simulink model "PLL_Sync_3_Phase"  (R2018a)
settings: Solver=ode23t  StartTime=0.0  StopTime=5  RelTol=1e-3
undefined symbols (not defined in the file): D1, Delta
libraries: powerlib x34, powerlib_meascontrol x4, simulink x3, dspswit3 x1
settings Model: Creator=samue  LastModifiedBy=samue

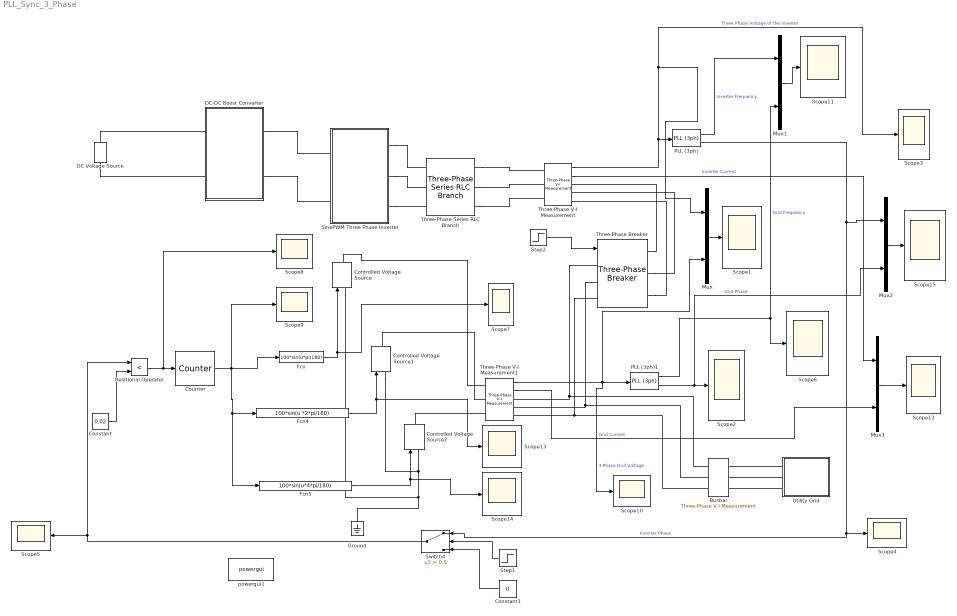
== system PLL_Sync_3_Phase ==
  Busbar : powerlib/Measurements/Three-Phase V-I Measurement  VoltageMeasurement=no  SetLabelV=off  LabelV=Vabc  Vpu=off  VpuLL=off  CurrentMeasurement=no  SetLabelI=off  LabelI=Iabc  Ipu=off  Pbase=100e6  Vbase=500e3  OutputType=Complex  PhasorSimulation=off  PSBequivalent=0
  Constant : Constant  Value=0.02
  Constant1 : Constant  Value=0
  Controlled Voltage Source : powerlib/Electrical Sources/Controlled Voltage Source  Initialize=on  Source_Type=AC  Amplitude=0  Phase=0  Frequency=60  Measurements=None
  Controlled Voltage Source1 : powerlib/Electrical Sources/Controlled Voltage Source  Initialize=on  Source_Type=AC  Amplitude=0  Phase=120  Frequency=60  Measurements=None
  Controlled Voltage Source2 : powerlib/Electrical Sources/Controlled Voltage Source  Initialize=on  Source_Type=AC  Amplitude=0  Phase=-120  Frequency=60  Measurements=None
  Counter : dspswit3/Counter  Direction=Up  CountEvent=Free running  CounterSize=User defined  MaxCount=360  InitialCount=0  Output=Count  HitValue=32  ResetInput=on  SamplesPerFrame=1  Ts=5e-5  CntDtype=double  HitDtype=Logical
  DC Voltage Source : powerlib/Electrical Sources/DC Voltage Source  Amplitude=100  Measurements=None
  DC-DC Boost Converter : Subsystem
  Fcn : Fcn  Expr=100*sin(u*pi/180)
  Fcn4 : Fcn  Expr=100*sin(u *2*pi/180)
  Fcn5 : Fcn  Expr=100*sin(u*4*pi/180)
  Ground : powerlib/Elements/Ground  LConnTagsString=a
  Mux{,1..3} (4 alike) : Mux  Inputs=2
  PLL (3ph) : powerlib_meascontrol/PLL/PLL (3ph)  Fmin=45  Par_Init=[0, 60]  ParK=[180, 3200, 1]  TcD=1e-4  MaxRateChangeFreq=12  FilterCutOffFreq=25  Ts=5e-5  AGC=on
  PLL (3ph)1 : powerlib_meascontrol/PLL/PLL (3ph)  Fmin=45  Par_Init=[0, 60]  ParK=[180, 3200, 1]  TcD=1e-4  MaxRateChangeFreq=12  FilterCutOffFreq=25  Ts=0  AGC=on
  Relational Operator : RelationalOperator  Operator=<  OutDataTypeStr=boolean  RndMeth=Simplest
  Scope{1..15} (15 alike) : Scope
  SinePWM Three Phase Inverter : Subsystem
  Step1 : Step  Time=0.06  SampleTime=0
  Step2 : Step  Time=0.1  SampleTime=0
  Switch4 : Switch  Criteria=u2 > Threshold  Threshold=0.5  RndMeth=Zero
  Three-Phase Series RLC Branch : powerlib/Elements/Three-Phase Series RLC Branch  LConnTagsString=A|B|C  RConnTagsString=A|B|C  BranchType=RLC  Resistance=1  Inductance=1e-3  Capacitance=1e-6  Measurements=None
  Three-Phase V-I Measurement : powerlib/Measurements/Three-Phase V-I Measurement  VoltageMeasurement=phase-to-ground  SetLabelV=off  LabelV=Vabc  Vpu=off  VpuLL=off  CurrentMeasurement=yes  SetLabelI=off  LabelI=Iabc  Ipu=off  Pbase=100e6  Vbase=500e3  OutputType=Complex  PhasorSimulation=off  PSBequivalent=0
  Three-Phase V-I Measurement1 : powerlib/Measurements/Three-Phase V-I Measurement  VoltageMeasurement=phase-to-ground  SetLabelV=off  LabelV=Vabc  Vpu=off  VpuLL=off  CurrentMeasurement=yes  SetLabelI=off  LabelI=Iabc  Ipu=off  Pbase=100e6  Vbase=500e3  OutputType=Complex  PhasorSimulation=off  PSBequivalent=0
  Three-Phase Breaker : powerlib/Elements/Three-Phase Breaker  InitialState=open  SwitchA=on  SwitchB=on  SwitchC=on  SwitchTimes="[1/60  5/60]"  External=on  BreakerResistance=0.01  SnubberResistance=1e6  SnubberCapacitance=inf  Measurements=None
  Utility Grid : Subsystem
  powergui1 : powerlib/powergui  Priority=1  SimulationMode=Discrete  SampleTime=5e-6  frequency=60  Iterations=50  frequencyindice=60  Pbase=100e6  ErrMax=1e-4  UnitsV=kV  UnitsW=MW  buscounter=0  FunctionMessages=off  echomessages=off  EnableUseOfTLC=off  CurrentSourceSwitches=off  DisableSnubberDevices=off  DisableRonSwitches=off  DisableVfSwitches=off  DisplayEquations=off  SolverType=Tustin/Backward Euler (TBE)  Interpol=off  ExternalGateDelay=off  methode=off  Ts=100  x0status=blocks  SPID=on  SwTol=0  HookPort=off  RestoreLinks=warning  ResistiveCurrentMeasurement=off  Frange=[0:2:500]  Ylog=off  Xlog=on  ShowGrid=off  save=off  variable=ZData  structure=0  ZoomFFT=off  StartTime=0.0  cycles=1  DisplayStyle=1  fundamental=60  FreqAxis=off  MaxFrequency=1000  frequencyindicesteady=1  RmsSteady=1  display=off
  wires:
  PLL (3ph)/2 -> Mux2/1, Switch4/1, Scope4/1  "Inverter Phase"
  Three-Phase V-I Measurement1/1 -> PLL (3ph)1/1, Mux/2, Scope10/1  "3 Phase Grid Voltage"
  Step1/1 -> Switch4/2
  Constant1/1 -> Switch4/3
  Step2/1 -> Three-Phase Breaker/1
  Three-Phase V-I Measurement/1 -> Scope3/1, Mux/1, PLL (3ph)/1  "Three Phase Voltage of the Inverter"
  Mux/1 -> Scope1/1
  PLL (3ph)1/2 -> Scope2/1, Mux2/2  "Grid Phase"
  PLL (3ph)1/1 -> Scope6/1, Mux1/2  "Grid Frequency"
  Counter/1 -> Scope9/1, Fcn/1, Fcn5/1, Fcn4/1
  Fcn/1 -> Scope7/1, Controlled Voltage Source/1
  Fcn5/1 -> Scope14/1, Controlled Voltage Source2/1
  Relational Operator/1 -> Scope8/1, Counter/1
  Constant/1 -> Relational Operator/2
  Switch4/1 -> Scope5/1, Relational Operator/1
  Fcn4/1 -> Scope13/1, Controlled Voltage Source1/1
  Mux1/1 -> Scope11/1
  PLL (3ph)/1 -> Mux1/1  "Inverter Frequency"
  Mux2/1 -> Scope15/1
  Three-Phase V-I Measurement/2 -> Mux3/1  "Inverter Current"
  Three-Phase V-I Measurement1/2 -> Mux3/2  "Grid Current"
  Mux3/1 -> Scope12/1
  connections:
  Three-Phase Breaker/RConn3 -- Three-Phase V-I Measurement/RConn3
  Three-Phase Breaker/RConn2 -- Three-Phase V-I Measurement/RConn2
  Three-Phase Breaker/RConn1 -- Three-Phase V-I Measurement/RConn1
  Three-Phase Breaker/LConn3 -- Busbar/LConn3 -- Three-Phase V-I Measurement1/RConn3
  Three-Phase Breaker/LConn2 -- Busbar/LConn2 -- Three-Phase V-I Measurement1/RConn2
  Three-Phase Breaker/LConn1 -- Busbar/LConn1 -- Three-Phase V-I Measurement1/RConn1
  Ground/LConn1 -- Controlled Voltage Source/LConn1 -- Controlled Voltage Source1/LConn1 -- Controlled Voltage Source2/LConn1
  Controlled Voltage Source/RConn1 -- Three-Phase V-I Measurement1/LConn1
  Controlled Voltage Source1/RConn1 -- Three-Phase V-I Measurement1/LConn2
  Controlled Voltage Source2/RConn1 -- Three-Phase V-I Measurement1/LConn3
  Three-Phase Series RLC Branch/RConn1 -- Three-Phase V-I Measurement/LConn1
  Three-Phase Series RLC Branch/RConn2 -- Three-Phase V-I Measurement/LConn2
  Three-Phase Series RLC Branch/RConn3 -- Three-Phase V-I Measurement/LConn3
  SinePWM Three Phase Inverter/RConn1 -- Three-Phase Series RLC Branch/LConn1
  SinePWM Three Phase Inverter/RConn2 -- Three-Phase Series RLC Branch/LConn2
  SinePWM Three Phase Inverter/RConn3 -- Three-Phase Series RLC Branch/LConn3
  Utility Grid/LConn1 -- Busbar/RConn1
  Utility Grid/LConn2 -- Busbar/RConn2
  Utility Grid/LConn3 -- Busbar/RConn3
  DC Voltage Source/LConn1 -- DC-DC Boost Converter/LConn2
  DC Voltage Source/RConn1 -- DC-DC Boost Converter/LConn1
  DC-DC Boost Converter/RConn1 -- SinePWM Three Phase Inverter/LConn1
  DC-DC Boost Converter/RConn2 -- SinePWM Three Phase Inverter/LConn2

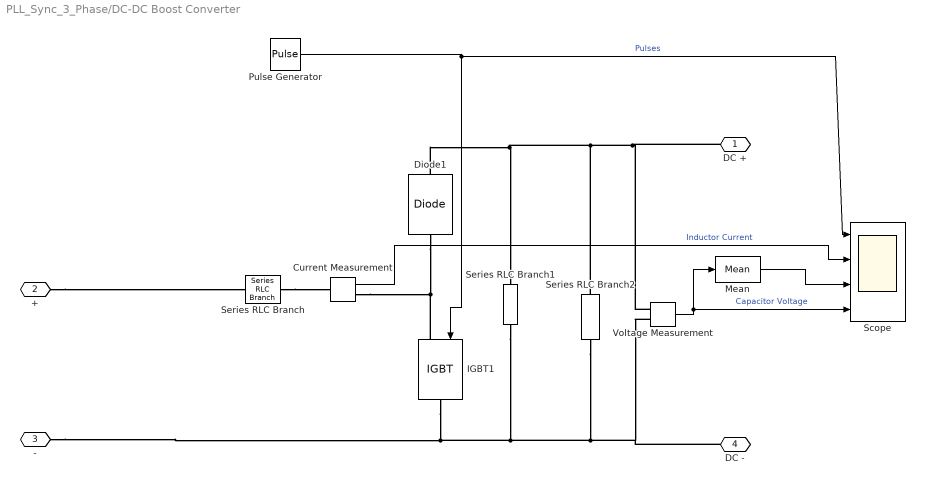
== system PLL_Sync_3_Phase/DC-DC Boost Converter ==
  Current Measurement : powerlib/Measurements/Current Measurement  PhasorSimulation=off  OutputType=Complex  PSBequivalent=0
  Diode1 : powerlib/Power Electronics/Diode  Ron=0.001  Lon=0  Vf=0.00001  IC=0  UseSnubber=0  Rs=5000000  Cs=250e-9  Measurements=off
  IGBT1 : powerlib/Power Electronics/IGBT  Ron=0.001  Lon=0  Vf=0.0001  Tf=1e-6  Tt=2e-6  IC=0  Rs=1e5  Cs=inf  Measurements=off
  Mean : powerlib_meascontrol/Measurements/Mean  Freq=60  Vinit=0  Ts=0
  Pulse Generator : DiscretePulseGenerator  PulseType=Time based  Period=1e-5  PulseWidth=50
  Scope : Scope  NumInputPorts=4
  Series RLC Branch : powerlib/Elements/Series RLC Branch  LConnTagsString=__new0  RConnTagsString=__new0  BranchType=L  Resistance=1  Inductance=200e-6  SetiL0=off  InitialCurrent=0  Capacitance=1e-6  Setx0=off  InitialVoltage=0  Measurements=None
  Series RLC Branch1 : powerlib/Elements/Series RLC Branch  LConnTagsString=__new0  RConnTagsString=__new0  BranchType=C  Resistance=1  Inductance=1e-3  SetiL0=off  InitialCurrent=0  Capacitance=100e-6  Setx0=off  InitialVoltage=0  Measurements=None
  Series RLC Branch2 : powerlib/Elements/Series RLC Branch  LConnTagsString=__new0  RConnTagsString=__new0  BranchType=R  Resistance=12  Inductance=1e-3  SetiL0=off  InitialCurrent=0  Capacitance=1e-6  Setx0=off  InitialVoltage=0  Measurements=None
  Voltage Measurement : powerlib/Measurements/Voltage Measurement  PhasorSimulation=off  OutputType=Complex  PSBequivalent=0
  DC + : PMIOPort  Side=Right
  + : PMIOPort  Port=2  Side=Left
  - : PMIOPort  Port=3  Side=Left
  DC - : PMIOPort  Port=4  Side=Right
  wires:
  Current Measurement/1 -> Scope/2  "Inductor Current"
  Voltage Measurement/1 -> Scope/4, Mean/1  "Capacitor Voltage"
  Pulse Generator/1 -> Scope/1, IGBT1/1  "Pulses"
  Mean/1 -> Scope/3
  connections:
  IGBT1/RConn1 -- Series RLC Branch1/RConn1 -- Voltage Measurement/LConn2 -- DC -/RConn1 -- Series RLC Branch2/RConn1 -- -/RConn1
  Voltage Measurement/LConn1 -- DC +/RConn1 -- Series RLC Branch2/LConn1 -- Diode1/RConn1 -- Series RLC Branch1/LConn1
  Diode1/LConn1 -- IGBT1/LConn1 -- Current Measurement/RConn1
  Series RLC Branch/RConn1 -- Current Measurement/LConn1
  +/RConn1 -- Series RLC Branch/LConn1

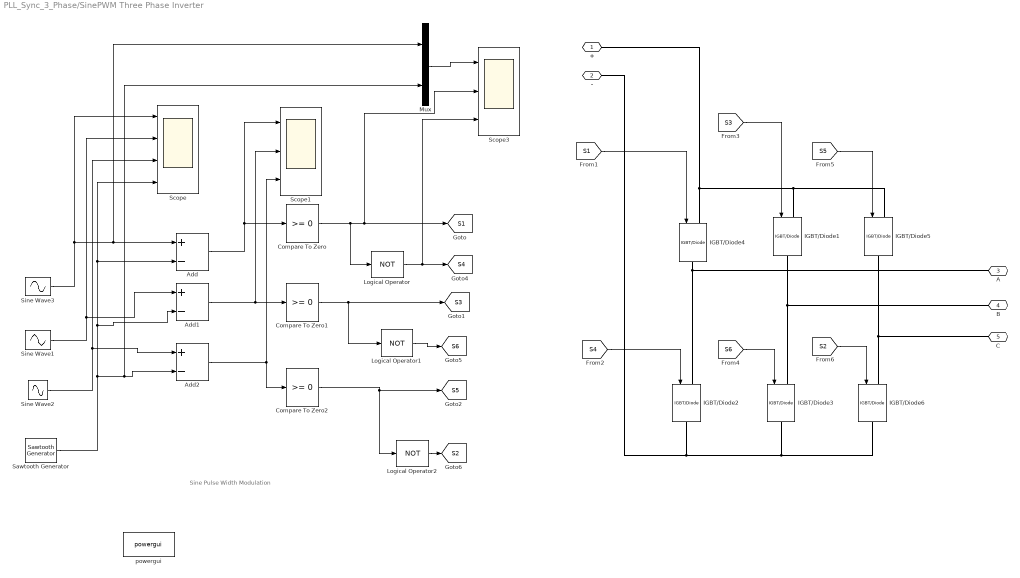
== system PLL_Sync_3_Phase/SinePWM Three Phase Inverter ==
  note: Sine Pulse Width Modulation
  Add : Sum  Inputs=+-
  Add1 : Sum  Inputs=+-
  Add2 : Sum  Inputs=+-
  Compare To Zero : simulink/Logic and Bit Operations/Compare To Zero  relop=>=  OutDataTypeStr=boolean
  Compare To Zero1 : simulink/Logic and Bit Operations/Compare To Zero  relop=>=  OutDataTypeStr=boolean
  Compare To Zero2 : simulink/Logic and Bit Operations/Compare To Zero  relop=>=  OutDataTypeStr=boolean
  IGBT/Diode{1..6} (6 alike) : powerlib/Power Electronics/IGBT//Diode  Ron=1e-3  Rs=1e5  Cs=inf  Measurements=off
  Logical Operator : Logic  Operator=NOT  AllPortsSameDT=off  OutDataTypeStr=boolean
  Logical Operator1 : Logic  Operator=NOT  AllPortsSameDT=off  OutDataTypeStr=boolean
  Logical Operator2 : Logic  Operator=NOT  AllPortsSameDT=off  OutDataTypeStr=boolean
  Mux : Mux  Inputs=2
  Sawtooth Generator : powerlib_meascontrol/Pulse & Signal Generators/Sawtooth Generator  Freq=1e3  Phase=180  Ts=0
      settings: SourceProductName=Simscape Power Systems
  Scope : Scope  NumInputPorts=4
  Scope1 : Scope  NumInputPorts=3
  Scope3 : Scope  NumInputPorts=3
  Sine Wave1 : Sin  Frequency=2*pi*60  Phase=(2*pi)/3  SampleTime=0
  Sine Wave2 : Sin  Frequency=2*pi*60  Phase=(-2*pi)/3  SampleTime=0
  Sine Wave3 : Sin  Frequency=2*pi*60  SampleTime=0
  powergui : powerlib/powergui  Priority=1  SimulationMode=Continuous  SampleTime=50e-6  frequency=60  Iterations=50  frequencyindice=0  Pbase=100e6  ErrMax=1e-4  UnitsV=kV  UnitsW=MW  buscounter=0  FunctionMessages=off  echomessages=off  EnableUseOfTLC=off  CurrentSourceSwitches=off  DisableSnubberDevices=off  DisableRonSwitches=off  DisableVfSwitches=off  DisplayEquations=off  SolverType=Tustin/Backward Euler (TBE)  Interpol=off  ExternalGateDelay=off  methode=off  Ts=100  x0status=blocks  SPID=on  SwTol=0  HookPort=off  RestoreLinks=warning  ResistiveCurrentMeasurement=off  Frange=[0:2:500]  Ylog=off  Xlog=on  ShowGrid=off  save=off  variable=ZData  structure=0  ZoomFFT=off  StartTime=0.0  cycles=1  DisplayStyle=1  fundamental=60  FreqAxis=off  MaxFrequency=1000  frequencyindicesteady=1  RmsSteady=1  display=off
  + : PMIOPort  Side=Left
  - : PMIOPort  Port=2  Side=Left
  A : PMIOPort  Port=3  Side=Right
  B : PMIOPort  Port=4  Side=Right
  C : PMIOPort  Port=5  Side=Right
  tag scope: S1=global, S2=global, S3=global, S4=global, S5=global, S6=global
  wires:
  Sawtooth Generator/1 -> Mux/2, Add2/2, Add1/2, Add/2, Scope/4
  Add/1 -> Scope1/1, Compare To Zero/1
  Add1/1 -> Compare To Zero1/1, Scope1/2
  Compare To Zero/1 -> [S1], Scope3/2, Logical Operator/1
  [S6] -> IGBT/Diode3/1
  Compare To Zero1/1 -> Logical Operator1/1, [S3]
  Sine Wave3/1 -> Mux/1, Add/1, Scope/1
  Sine Wave2/1 -> Add2/1, Scope/3
  Mux/1 -> Scope3/1
  Compare To Zero2/1 -> Logical Operator2/1, [S5]
  [S2] -> IGBT/Diode6/1
  [S1] -> IGBT/Diode4/1
  [S3] -> IGBT/Diode1/1
  [S4] -> IGBT/Diode2/1
  [S5] -> IGBT/Diode5/1
  Add2/1 -> Compare To Zero2/1, Scope1/3
  Sine Wave1/1 -> Add1/1, Scope/2
  Logical Operator2/1 -> [S2]
  Logical Operator1/1 -> [S6]
  Logical Operator/1 -> Scope3/3, [S4]
  connections:
  IGBT/Diode6/LConn1 -- C/RConn1 -- IGBT/Diode5/RConn1
  IGBT/Diode4/RConn1 -- IGBT/Diode2/LConn1 -- A/RConn1
  IGBT/Diode4/LConn1 -- +/RConn1 -- IGBT/Diode5/LConn1 -- IGBT/Diode1/LConn1
  IGBT/Diode6/RConn1 -- -/RConn1 -- IGBT/Diode2/RConn1 -- IGBT/Diode3/RConn1
  IGBT/Diode3/LConn1 -- B/RConn1 -- IGBT/Diode1/RConn1

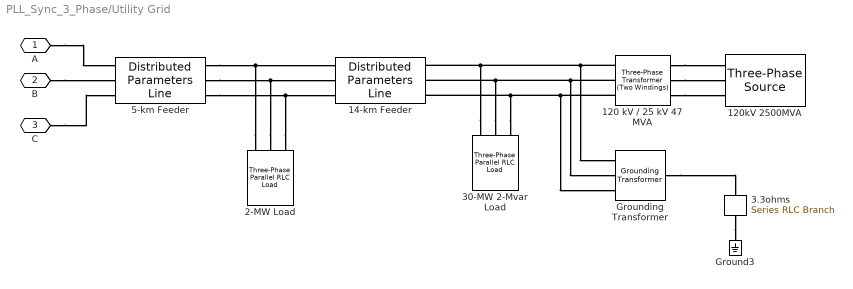
== system PLL_Sync_3_Phase/Utility Grid ==
  120 kV / 25 kV 47 MVA : powerlib/Elements/Three-Phase Transformer (Two Windings)  Winding1Connection=Yg  Winding2Connection=Delta (D1)  CoreType=Three single-phase transformers  SetSaturation=off  Hysteresis=off  DataFile='basic_model'  SetInitialFlux=off  Measurements=None  UNITS=pu  NominalPower=[47e6 60 ]  Winding1="[ 120e3  0.08/30   0.08 ]"  Winding2="[ 25e3  0.08/30  0.08]"  Rm=500  Lm=500  L0=0.5  Saturation="[ 0,0  ;  0.005,1.2  ;  1.0,1.4 ]"  InitialFluxes=[ 0.8 , -0.8 , 0.7 ]  MoreParameters=off  BreakLoop=off  DataType=off  TransfoNumber=0
  120kV 2500MVA : powerlib/Electrical Sources/Three-Phase Source  InternalConnection=Yg  VoltagePhases=off  Voltage=120e3  PhaseAngle=0  Voltage_phases=[25e3 25e3 25e3]/sqrt(3)  PhaseAngles_phases=[0 -120 +120]  Frequency=60  NonIdealSource=on  SpecifyImpedance=on  Resistance=0.8929  Inductance=16.58e-3  ShortCircuitLevel=2500e6  BaseVoltage=120e3  XRratio=7  BusType=swing  Pref=0  Qref=0  Prefabc=[10e3, 10e3, 10e3]  Qrefabc=[0, 0, 0]  Qmin=-inf  Qmax=inf
  14-km Feeder : powerlib/Elements/Distributed Parameters Line  Phases=3  Frequency=60  Resistance=[0.1153 0.413]  Inductance=[1.05e-3 3.32e-3]  Capacitance=[11.33e-009 5.01e-009]  Length=14  x1=[-6e-05 1.37030160408931e-09 -837.178421983371 -4898.29413559374;-5.5e-05 1.36683884590095e-09 -827.943873256933 -4899.86347684942;-5e-05 1.36337123125689e-09 -818.706382799107 -4901.41540861316;-4.5e-05 1.35989877247778e-09 -809.46598343122 -4902.94992537087;-4e-05 1.35642148190145e-09 -800.222707984933 -4904.46702167032;-3.5e-05 1.35293937188291e-09 -790.976589302125 -4905.96669212118;-3e-05 1.3494524547943e-09 -781.727660234781 -4907.44893139504;-2.5e-05 1.34596074302483e-09 -772.475953644866 -4908.91373422541;-2e-05 1.34246424898074e-09 -763.221502404218 -4910.36109540777;-1.5e-05 1.33896298508529e-09 -753.964339394426 -4911.79100979957;-1e-05 1.33545696377866e-09 -744.704497506712 -4913.20347232023;-5e-06 1.33194619751794e-09 -735.442009641819 -4914.59847795121]  x2=[-6e-05 5.08712230264926e-09 -3097.87964222434 -18651.9887557223;-5.5e-05 5.07453697378858e-09 -3062.7159890635 -18657.7949820346;-5e-05 5.06193361481116e-09 -3027.54145389961 -18663.5349161465;-4.5e-05 5.04931227049744e-09 -2992.35616170978 -18669.2085376637;-4e-05 5.03667298569178e-09 -2957.16023750934 -18674.8158264276;-3.5e-05 5.02401580530226e-09 -2921.95380635141 -18680.3567625152;-3e-05 5.01134077430056e-09 -2886.73699332641 -18685.8313262391;-2.5e-05 4.99864793772179e-09 -2851.50992356168 -18691.239498148;-2e-05 4.98593734066431e-09 -2816.27272222099 -18696.5812590262;-1.5e-05 4.9732090282896e-09 -2781.02551450411 -18701.8565898943;-1e-05 4.96046304582206e-09 -2745.76842564636 -18707.0654720087;-5e-06 4.94769943854889e-09 -2710.50158091816 -18712.2078868619]  x3=[-6e-05 3.12910261542347e-10 -2393.9333377164 -305.532683111771;-5.5e-05 3.1311058091873e-10 -2393.35316962759 -310.044595684322;-5e-05 3.13309787795519e-10 -2392.76449781966 -314.555406650896;-4.5e-05 3.13507881464919e-10 -2392.1673243842 -319.065099984328;-4e-05 3.13704861223094e-10 -2391.561651443 -323.573659661422;-3.5e-05 3.13900726370161e-10 -2390.94748114805 -328.081069663011;-3e-05 3.14095476210203e-10 -2390.32481568154 -332.587313974013;-2.5e-05 3.14289110051261e-10 -2389.69365725583 -337.092376583486;-2e-05 3.14481627205343e-10 -2389.05400811345 -341.596241484688;-1.5e-05 3.14673026988426e-10 -2388.40587052713 -346.098892675133;-1e-05 3.14863308720454e-10 -2387.74924679973 -350.600314156646;-5e-06 3.15052471725347e-10 -2387.08413926427 -355.100489935423]  x4=[-6e-05 -3.04931956519203e-10 2380.3561252703 228.597013568549;-5.5e-05 -3.05150318536322e-10 2379.92100153645 233.08347039212;-5e-05 -3.05367596337108e-10 2379.47742180874 237.569099056944;-4.5e-05 -3.05583789149561e-10 2379.02538766323 242.053883625328;-4e-05 -3.05798896205536e-10 2378.56490070603 246.537808162581;-3.5e-05 -3.06012916740745e-10 2378.09596257327 251.020856737063;-3e-05 -3.06225849994761e-10 2377.61857493111 255.503013420251;-2.5e-05 -3.06437695211021e-10 2377.13273947575 259.984262286788;-2e-05 -3.06648451636826e-10 2376.63845793338 264.464587414544;-1.5e-05 -3.06858118523346e-10 2376.1357320602 268.943972884669;-1e-05 -3.07066695125624e-10 2375.62456364245 273.422402781655;-5e-06 -3.07274180702576e-10 2375.10495449632 277.899861193387]  x5=5.70973484498186e-05  V1=ones(3,3)  V2=ones(3,3)  I1=ones(3,3)  I2=ones(3,3)  nHarmo=1  Measurements=None
      settings: SourceProductName=Simscape Power Systems
  2-MW Load : powerlib/Elements/Three-Phase Parallel RLC Load  LConnTagsString=A|B|C  Configuration=Y (grounded)  NominalVoltage=25e3  Vabc=[1e3 1e3 1e3]  Vabcp=[1e3 1e3 1e3]  NominalFrequency=60  UnbalancedPower=off  ActivePower=2e6  InductivePower=0  CapacitivePower=0  Pabc=[10e3 9e3 11e3]  QLabc=[100 90 110]  QCabc=[100 90 110]  Pabcp=[10e3 9e3 11e3]  QLabcp=[100 90 110]  QCabcp=[100 90 110]  Measurements=None  LoadType=constant Z
  "3.3ohms " : powerlib/Elements/Series RLC Branch  LConnTagsString=__new0  RConnTagsString=__new0  BranchType=R  Resistance=3.3  Inductance=[]  SetiL0=off  InitialCurrent=0  Capacitance=[]  Setx0=off  InitialVoltage=0  Measurements=None
  30-MW 2-Mvar Load : powerlib/Elements/Three-Phase Parallel RLC Load  LConnTagsString=A|B|C  Configuration=Y (grounded)  NominalVoltage=25e3  Vabc=[1e3 1e3 1e3]  Vabcp=[1e3 1e3 1e3]  NominalFrequency=60  UnbalancedPower=off  ActivePower=30e6  InductivePower=2e6  CapacitivePower=0  Pabc=[10e3 9e3 11e3]  QLabc=[100 90 110]  QCabc=[100 90 110]  Pabcp=[10e3 9e3 11e3]  QLabcp=[100 90 110]  QCabcp=[100 90 110]  Measurements=None  LoadType=constant Z
  5-km Feeder : powerlib/Elements/Distributed Parameters Line  Phases=3  Frequency=60  Resistance=[0.1153 0.413]  Inductance=[1.05e-3 3.32e-3]  Capacitance=[11.33e-009 5.01e-009]  Length=5  x1=[-2.5e-05 0 0 0;-2e-05 0 0 0;-1.5e-05 0 0 0;-1e-05 0 0 0;-5e-06 0 0 0]  x2=[-2.5e-05 1.34584545405026e-09 0 0;-2e-05 1.34234927961883e-09 -763.221502404218 -4910.36109540777;-1.5e-05 1.33884833574454e-09 -753.964339394426 -4911.79100979957;-1e-05 1.33534263486641e-09 -744.704497506712 -4913.20347232023;-5e-06 1.33183218944042e-09 -735.442009641819 -4914.59847795121]  x3=[-2.5e-05 3.30735135908525e-10 0 0;-2e-05 3.30933481340074e-10 -2388.24027947955 -310.379138748703;-1.5e-05 3.31130650946255e-10 -2387.65098615636 -314.880311555783;-1e-05 3.31326644026514e-10 -2387.05320937425 -319.380365575314;-5e-06 3.31521459884476e-10 -2386.44695125713 -323.879284818352]  x4=[-2.5e-05 -3.29438575094476e-10 0 0;-2e-05 -3.29640752377991e-10 2385.68435713408 294.280195880359;-1.5e-05 -3.29841758429277e-10 2385.12541412599 298.776579490401;-1e-05 -3.30041592534149e-10 2384.55799663246 303.271901530365;-5e-06 -3.30240253982584e-10 2383.98210666956 307.766146028118]  x5=2.03919101606495e-05  V1=ones(3,3)  V2=ones(3,3)  I1=ones(3,3)  I2=ones(3,3)  nHarmo=1  Measurements=None
      settings: SourceProductName=Simscape Power Systems
  Ground3 : powerlib/Elements/Ground  LConnTagsString=a
  "Grounding Transformer " : powerlib/Elements/Grounding Transformer   UNITS=pu  NominalPower="[100e6   60]"  NominalVoltage=25e3  ZeroSequenceImpedance_pu=[0.025 0.75]  MagnetizationBranch_pu=[500 500]  ZeroSequenceImpedance_SI=[0.052083 589.05]  MagnetizationBranch_SI=[1041.7 3.927e+005]  Measurements=None
      settings: SourceProductName=Simscape Power Systems  SourceProductBaseCode=PS
  A : PMIOPort  Side=Left
  B : PMIOPort  Port=2  Side=Left
  C : PMIOPort  Port=3  Side=Left
  connections:
  30-MW 2-Mvar Load/LConn2 -- 14-km Feeder/RConn2 -- 120 kV / 25 kV 47 MVA/RConn2 -- "Grounding Transformer "/LConn2
  "3.3ohms "/RConn1 -- Ground3/LConn1
  30-MW 2-Mvar Load/LConn3 -- 14-km Feeder/RConn3 -- 120 kV / 25 kV 47 MVA/RConn3 -- "Grounding Transformer "/LConn3
  2-MW Load/LConn1 -- 5-km Feeder/RConn1 -- 14-km Feeder/LConn1
  30-MW 2-Mvar Load/LConn1 -- 14-km Feeder/RConn1 -- 120 kV / 25 kV 47 MVA/RConn1 -- "Grounding Transformer "/LConn1
  2-MW Load/LConn3 -- 5-km Feeder/RConn3 -- 14-km Feeder/LConn3
  A/RConn1 -- 5-km Feeder/LConn1
  2-MW Load/LConn2 -- 5-km Feeder/RConn2 -- 14-km Feeder/LConn2
  120 kV / 25 kV 47 MVA/LConn2 -- 120kV 2500MVA/RConn2
  "Grounding Transformer "/RConn1 -- "3.3ohms "/LConn1
  120 kV / 25 kV 47 MVA/LConn1 -- 120kV 2500MVA/RConn1
  C/RConn1 -- 5-km Feeder/LConn3
  120 kV / 25 kV 47 MVA/LConn3 -- 120kV 2500MVA/RConn3
  B/RConn1 -- 5-km Feeder/LConn2
